simulink library "TYPEB_MASTER"  (Simulink 8.8)
settings: Solver=ode45  StartTime=0.0  StopTime=10.0  RelTol=1e-3  EnableMultiTasking=on
libraries: cdsEpicsOut x65, cdsTP x48, cdsFilt x34, cdsEpicsStringIn x29, cdsFiltCtrl x27, cdsRms x24, STATE_BIO_MASTER x15, cdsEpicsBinIn x14, cdsBit2Word x12, GAS_MASTER x9, cdsWord2Bit x5, cdsDacKill x4
(part 3 of 6)

== system TYPEB_MASTER/TYPEB_MASTER/TM_OSEM/DAMP ==
  LONG_In : Inport
  PITCH_In : Inport  Port=2
  YAW_In : Inport  Port=3
  Ground{1..2,6,8..9,12} (6 alike) : Ground
  L : cdsFiltCtrl/IIR FM with control  Tag=cdsFiltCtrl  Description=|
      | cdsFiltCntrl is the standard IIR filter module (exactly the same as cdsFilt) but with added control data output 'Ctrl'. Filter module digital signal output appears on the first output, which is called 'Val'. 'Ctrl' output has a bit pattern encoding the state of filter's on/off switches (FM1 through FM10). The bit values are:
      |                                                                                                                                                                                                                                                                                                                                       
      | module 	hex	dec                                                                                                                                                                                                                                                                                                                       
      | -----------------------                                                                                                                                                                                                                                                                                                               
      | FM1	0x20                    32                                                                                                                                                                                                                                                                                                        
      | FM2	0x80                     128                                                                                                                                                                                                                                                                                                      
      | FM3	0x200                   512                                                                                                                                                                                                                                                                                                       
      | FM4	0x800                   2048                                                                                                                                                                                                                                                                                                      
      | FM5	0x2000                 8192                                                                                                                                                                                                                                                                                                       
      | FM6	0x8000                 32768                                                                                                                                                                                                                                                                                                      
      | FM7	0x20000                131072                                                                                                                                                                                                                                                                                                     
      | FM8	0x80000                 524288                                                                                                                                                                                                                                                                                                    
      | FM9	0x200000               2097152                                                                                                                                                                                                                                                                                                    
      | FM10	0x800000               8388608                                                                                                                                                                                                                                                                                                   
      |                                                                                                                                                                                                                                                                                                                                       
      | This bit data can be used to drive some other switches or it can be output using a binary I/O module.
      settings: AttributesFormatString=%<Tag>
  P : cdsFiltCtrl/IIR FM with control  Tag=cdsFiltCtrl  Description=|
      | cdsFiltCntrl is the standard IIR filter module (exactly the same as cdsFilt) but with added control data output 'Ctrl'. Filter module digital signal output appears on the first output, which is called 'Val'. 'Ctrl' output has a bit pattern encoding the state of filter's on/off switches (FM1 through FM10). The bit values are:
      |                                                                                                                                                                                                                                                                                                                                       
      | module 	hex	dec                                                                                                                                                                                                                                                                                                                       
      | -----------------------                                                                                                                                                                                                                                                                                                               
      | FM1	0x20                    32                                                                                                                                                                                                                                                                                                        
      | FM2	0x80                     128                                                                                                                                                                                                                                                                                                      
      | FM3	0x200                   512                                                                                                                                                                                                                                                                                                       
      | FM4	0x800                   2048                                                                                                                                                                                                                                                                                                      
      | FM5	0x2000                 8192                                                                                                                                                                                                                                                                                                       
      | FM6	0x8000                 32768                                                                                                                                                                                                                                                                                                      
      | FM7	0x20000                131072                                                                                                                                                                                                                                                                                                     
      | FM8	0x80000                 524288                                                                                                                                                                                                                                                                                                    
      | FM9	0x200000               2097152                                                                                                                                                                                                                                                                                                    
      | FM10	0x800000               8388608                                                                                                                                                                                                                                                                                                   
      |                                                                                                                                                                                                                                                                                                                                       
      | This bit data can be used to drive some other switches or it can be output using a binary I/O module.
      settings: AttributesFormatString=%<Tag>
  Terminator{1..3,6..8} (6 alike) : Terminator
  Y : cdsFiltCtrl/IIR FM with control  Tag=cdsFiltCtrl  Description=|
      | cdsFiltCntrl is the standard IIR filter module (exactly the same as cdsFilt) but with added control data output 'Ctrl'. Filter module digital signal output appears on the first output, which is called 'Val'. 'Ctrl' output has a bit pattern encoding the state of filter's on/off switches (FM1 through FM10). The bit values are:
      |                                                                                                                                                                                                                                                                                                                                       
      | module 	hex	dec                                                                                                                                                                                                                                                                                                                       
      | -----------------------                                                                                                                                                                                                                                                                                                               
      | FM1	0x20                    32                                                                                                                                                                                                                                                                                                        
      | FM2	0x80                     128                                                                                                                                                                                                                                                                                                      
      | FM3	0x200                   512                                                                                                                                                                                                                                                                                                       
      | FM4	0x800                   2048                                                                                                                                                                                                                                                                                                      
      | FM5	0x2000                 8192                                                                                                                                                                                                                                                                                                       
      | FM6	0x8000                 32768                                                                                                                                                                                                                                                                                                      
      | FM7	0x20000                131072                                                                                                                                                                                                                                                                                                     
      | FM8	0x80000                 524288                                                                                                                                                                                                                                                                                                    
      | FM9	0x200000               2097152                                                                                                                                                                                                                                                                                                    
      | FM10	0x800000               8388608                                                                                                                                                                                                                                                                                                   
      |                                                                                                                                                                                                                                                                                                                                       
      | This bit data can be used to drive some other switches or it can be output using a binary I/O module.
      settings: AttributesFormatString=%<Tag>
  wires:
  Ground12/1 -> Y/3
  Ground9/1 -> P/3
  Ground8/1 -> L/3
  PITCH_In/1 -> P/1
  YAW_In/1 -> Y/1
  LONG_In/1 -> L/1
  Ground2/1 -> Y/2
  Ground1/1 -> P/2
  Ground6/1 -> L/2
  L/1 -> Terminator6/1
  L/2 -> Terminator1/1
  P/1 -> Terminator3/1
  P/2 -> Terminator2/1
  Y/1 -> Terminator8/1
  Y/2 -> Terminator7/1

== system TYPEB_MASTER/TYPEB_MASTER/TM_OSEM/INF ==
  H1_In : Inport
  H2_In : Inport  Port=2
  H3_In : Inport  Port=3
  H4_In : Inport  Port=4
  H1 : cdsFilt/Subsystem  Tag=cdsFilt  Description=|
      | Purpose:                                                                                                                                                                                                                                  
      | Standard CDS IIR filter module.                                                                                                                                                                                                           
      |                                                                                                                                                                                                                                           
      | Operation:                                                                                                                                                                                                                                
      | Consists of 10 second order section IIR filters, plus a ramped gain stage. In FE code, also provides pre-defined test points and excitation channel inputs. The filter coefficients are defined in the LIGO system using the 'foton' tool.
      |                                                                                                                                                                                                                                           
      | Usage:                                                                                                                                                                                                                                    
      | Name the part with the desired filter module name.
      settings: AttributesFormatString=%<Tag>
  H2 : cdsFilt/Subsystem  Tag=cdsFilt  Description=|
      | Purpose:                                                                                                                                                                                                                                  
      | Standard CDS IIR filter module.                                                                                                                                                                                                           
      |                                                                                                                                                                                                                                           
      | Operation:                                                                                                                                                                                                                                
      | Consists of 10 second order section IIR filters, plus a ramped gain stage. In FE code, also provides pre-defined test points and excitation channel inputs. The filter coefficients are defined in the LIGO system using the 'foton' tool.
      |                                                                                                                                                                                                                                           
      | Usage:                                                                                                                                                                                                                                    
      | Name the part with the desired filter module name.
      settings: AttributesFormatString=%<Tag>
  H3 : cdsFilt/Subsystem  Tag=cdsFilt  Description=|
      | Purpose:                                                                                                                                                                                                                                  
      | Standard CDS IIR filter module.                                                                                                                                                                                                           
      |                                                                                                                                                                                                                                           
      | Operation:                                                                                                                                                                                                                                
      | Consists of 10 second order section IIR filters, plus a ramped gain stage. In FE code, also provides pre-defined test points and excitation channel inputs. The filter coefficients are defined in the LIGO system using the 'foton' tool.
      |                                                                                                                                                                                                                                           
      | Usage:                                                                                                                                                                                                                                    
      | Name the part with the desired filter module name.
      settings: AttributesFormatString=%<Tag>
  H4 : cdsFilt/Subsystem  Tag=cdsFilt  Description=|
      | Purpose:                                                                                                                                                                                                                                  
      | Standard CDS IIR filter module.                                                                                                                                                                                                           
      |                                                                                                                                                                                                                                           
      | Operation:                                                                                                                                                                                                                                
      | Consists of 10 second order section IIR filters, plus a ramped gain stage. In FE code, also provides pre-defined test points and excitation channel inputs. The filter coefficients are defined in the LIGO system using the 'foton' tool.
      |                                                                                                                                                                                                                                           
      | Usage:                                                                                                                                                                                                                                    
      | Name the part with the desired filter module name.
      settings: AttributesFormatString=%<Tag>
  H4_Out : Outport
  H1_Out : Outport  Port=2
  H2_Out : Outport  Port=3
  H3_Out : Outport  Port=4
  wires:
  H4/1 -> H4_Out/1
  H4_In/1 -> H4/1
  H1/1 -> H1_Out/1
  H2/1 -> H2_Out/1
  H3/1 -> H3_Out/1
  H1_In/1 -> H1/1
  H2_In/1 -> H2/1
  H3_In/1 -> H3/1

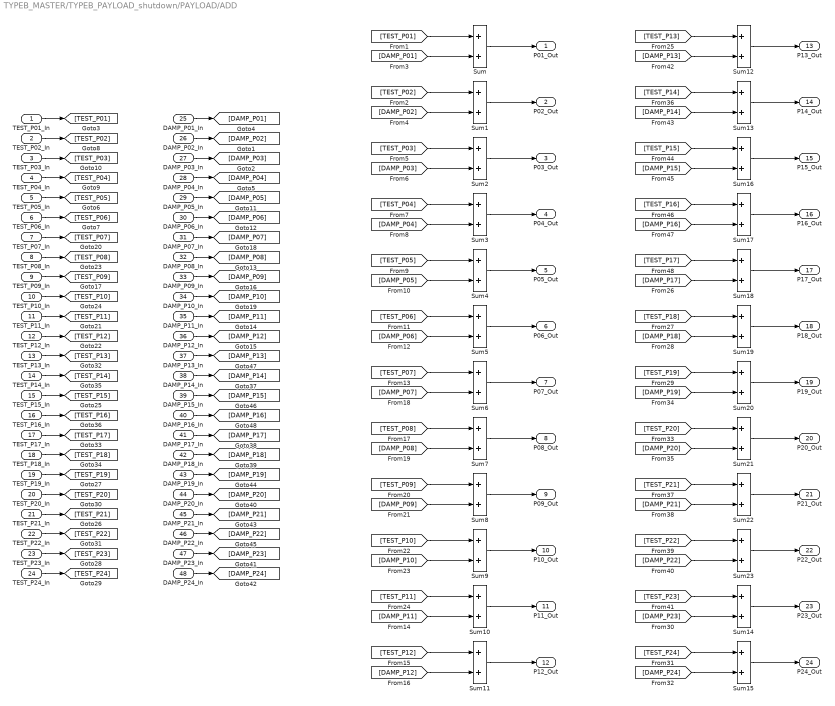
== system TYPEB_MASTER/TYPEB_PAYLOAD_shutdown/PAYLOAD/ADD ==
  TEST_P01_In : Inport
  TEST_P02_In : Inport  Port=2
  TEST_P03_In : Inport  Port=3
  TEST_P04_In : Inport  Port=4
  TEST_P05_In : Inport  Port=5
  TEST_P06_In : Inport  Port=6
  TEST_P07_In : Inport  Port=7
  TEST_P08_In : Inport  Port=8
  TEST_P09_In : Inport  Port=9
  TEST_P10_In : Inport  Port=10
  TEST_P11_In : Inport  Port=11
  TEST_P12_In : Inport  Port=12
  TEST_P13_In : Inport  Port=13
  TEST_P14_In : Inport  Port=14
  TEST_P15_In : Inport  Port=15
  TEST_P16_In : Inport  Port=16
  TEST_P17_In : Inport  Port=17
  TEST_P18_In : Inport  Port=18
  TEST_P19_In : Inport  Port=19
  TEST_P20_In : Inport  Port=20
  TEST_P21_In : Inport  Port=21
  TEST_P22_In : Inport  Port=22
  TEST_P23_In : Inport  Port=23
  TEST_P24_In : Inport  Port=24
  DAMP_P01_In : Inport  Port=25
  DAMP_P02_In : Inport  Port=26
  DAMP_P03_In : Inport  Port=27
  DAMP_P04_In : Inport  Port=28
  DAMP_P05_In : Inport  Port=29
  DAMP_P06_In : Inport  Port=30
  DAMP_P07_In : Inport  Port=31
  DAMP_P08_In : Inport  Port=32
  DAMP_P09_In : Inport  Port=33
  DAMP_P10_In : Inport  Port=34
  DAMP_P11_In : Inport  Port=35
  DAMP_P12_In : Inport  Port=36
  DAMP_P13_In : Inport  Port=37
  DAMP_P14_In : Inport  Port=38
  DAMP_P15_In : Inport  Port=39
  DAMP_P16_In : Inport  Port=40
  DAMP_P17_In : Inport  Port=41
  DAMP_P18_In : Inport  Port=42
  DAMP_P19_In : Inport  Port=43
  DAMP_P20_In : Inport  Port=44
  DAMP_P21_In : Inport  Port=45
  DAMP_P22_In : Inport  Port=46
  DAMP_P23_In : Inport  Port=47
  DAMP_P24_In : Inport  Port=48
  Sum{,1..23} (24 alike) : Sum
  P01_Out : Outport
  P02_Out : Outport  Port=2
  P03_Out : Outport  Port=3
  P04_Out : Outport  Port=4
  P05_Out : Outport  Port=5
  P06_Out : Outport  Port=6
  P07_Out : Outport  Port=7
  P08_Out : Outport  Port=8
  P09_Out : Outport  Port=9
  P10_Out : Outport  Port=10
  P11_Out : Outport  Port=11
  P12_Out : Outport  Port=12
  P13_Out : Outport  Port=13
  P14_Out : Outport  Port=14
  P15_Out : Outport  Port=15
  P16_Out : Outport  Port=16
  P17_Out : Outport  Port=17
  P18_Out : Outport  Port=18
  P19_Out : Outport  Port=19
  P20_Out : Outport  Port=20
  P21_Out : Outport  Port=21
  P22_Out : Outport  Port=22
  P23_Out : Outport  Port=23
  P24_Out : Outport  Port=24
  wires:
  Sum15/1 -> P24_Out/1
  [DAMP_P24] -> Sum15/2
  [TEST_P24] -> Sum15/1
  Sum14/1 -> P23_Out/1
  [TEST_P23] -> Sum14/1
  [DAMP_P23] -> Sum14/2
  Sum23/1 -> P22_Out/1
  [TEST_P22] -> Sum23/1
  [DAMP_P22] -> Sum23/2
  Sum22/1 -> P21_Out/1
  [TEST_P21] -> Sum22/1
  [DAMP_P21] -> Sum22/2
  Sum21/1 -> P20_Out/1
  [TEST_P20] -> Sum21/1
  [DAMP_P20] -> Sum21/2
  Sum20/1 -> P19_Out/1
  [TEST_P19] -> Sum20/1
  [DAMP_P19] -> Sum20/2
  Sum19/1 -> P18_Out/1
  [TEST_P18] -> Sum19/1
  [DAMP_P18] -> Sum19/2
  Sum18/1 -> P17_Out/1
  [TEST_P17] -> Sum18/1
  [DAMP_P17] -> Sum18/2
  Sum17/1 -> P16_Out/1
  [TEST_P16] -> Sum17/1
  [DAMP_P16] -> Sum17/2
  Sum16/1 -> P15_Out/1
  [TEST_P15] -> Sum16/1
  [DAMP_P15] -> Sum16/2
  Sum13/1 -> P14_Out/1
  [TEST_P14] -> Sum13/1
  [DAMP_P14] -> Sum13/2
  Sum12/1 -> P13_Out/1
  [TEST_P13] -> Sum12/1
  [DAMP_P13] -> Sum12/2
  DAMP_P24_In/1 -> [DAMP_P24]
  DAMP_P22_In/1 -> [DAMP_P22]
  DAMP_P23_In/1 -> [DAMP_P23]
  DAMP_P21_In/1 -> [DAMP_P21]
  DAMP_P19_In/1 -> [DAMP_P19]
  DAMP_P20_In/1 -> [DAMP_P20]
  DAMP_P18_In/1 -> [DAMP_P18]
  DAMP_P16_In/1 -> [DAMP_P16]
  DAMP_P17_In/1 -> [DAMP_P17]
  DAMP_P15_In/1 -> [DAMP_P15]
  DAMP_P13_In/1 -> [DAMP_P13]
  DAMP_P14_In/1 -> [DAMP_P14]
  TEST_P24_In/1 -> [TEST_P24]
  TEST_P23_In/1 -> [TEST_P23]
  TEST_P22_In/1 -> [TEST_P22]
  TEST_P21_In/1 -> [TEST_P21]
  TEST_P20_In/1 -> [TEST_P20]
  TEST_P19_In/1 -> [TEST_P19]
  TEST_P18_In/1 -> [TEST_P18]
  TEST_P17_In/1 -> [TEST_P17]
  TEST_P16_In/1 -> [TEST_P16]
  TEST_P15_In/1 -> [TEST_P15]
  TEST_P14_In/1 -> [TEST_P14]
  TEST_P13_In/1 -> [TEST_P13]
  Sum11/1 -> P12_Out/1
  [TEST_P12] -> Sum11/1
  [DAMP_P12] -> Sum11/2
  Sum10/1 -> P11_Out/1
  [TEST_P11] -> Sum10/1
  [DAMP_P11] -> Sum10/2
  Sum9/1 -> P10_Out/1
  [TEST_P10] -> Sum9/1
  [DAMP_P10] -> Sum9/2
  Sum8/1 -> P09_Out/1
  [TEST_P09] -> Sum8/1
  [DAMP_P09] -> Sum8/2
  Sum7/1 -> P08_Out/1
  [TEST_P08] -> Sum7/1
  [DAMP_P08] -> Sum7/2
  Sum6/1 -> P07_Out/1
  [TEST_P07] -> Sum6/1
  [DAMP_P07] -> Sum6/2
  Sum5/1 -> P06_Out/1
  [TEST_P06] -> Sum5/1
  [DAMP_P06] -> Sum5/2
  Sum4/1 -> P05_Out/1
  [TEST_P05] -> Sum4/1
  [DAMP_P05] -> Sum4/2
  Sum3/1 -> P04_Out/1
  [TEST_P04] -> Sum3/1
  [DAMP_P04] -> Sum3/2
  Sum2/1 -> P03_Out/1
  [TEST_P03] -> Sum2/1
  [DAMP_P03] -> Sum2/2
  Sum1/1 -> P02_Out/1
  [TEST_P02] -> Sum1/1
  [DAMP_P02] -> Sum1/2
  TEST_P12_In/1 -> [TEST_P12]
  TEST_P11_In/1 -> [TEST_P11]
  TEST_P10_In/1 -> [TEST_P10]
  TEST_P09_In/1 -> [TEST_P09]
  TEST_P08_In/1 -> [TEST_P08]
  TEST_P07_In/1 -> [TEST_P07]
  DAMP_P12_In/1 -> [DAMP_P12]
  DAMP_P10_In/1 -> [DAMP_P10]
  DAMP_P11_In/1 -> [DAMP_P11]
  DAMP_P09_In/1 -> [DAMP_P09]
  DAMP_P07_In/1 -> [DAMP_P07]
  DAMP_P08_In/1 -> [DAMP_P08]
  DAMP_P06_In/1 -> [DAMP_P06]
  DAMP_P04_In/1 -> [DAMP_P04]
  DAMP_P05_In/1 -> [DAMP_P05]
  TEST_P06_In/1 -> [TEST_P06]
  TEST_P05_In/1 -> [TEST_P05]
  TEST_P04_In/1 -> [TEST_P04]
  TEST_P03_In/1 -> [TEST_P03]
  TEST_P02_In/1 -> [TEST_P02]
  TEST_P01_In/1 -> [TEST_P01]
  DAMP_P03_In/1 -> [DAMP_P03]
  Sum/1 -> P01_Out/1
  [TEST_P01] -> Sum/1
  [DAMP_P01] -> Sum/2
  DAMP_P01_In/1 -> [DAMP_P01]
  DAMP_P02_In/1 -> [DAMP_P02]
